simulink model "parcial2"  (R2020b)
settings: Solver=VariableStepAuto  StartTime=0.0  StopTime=30  MaxStep=1e-2  RelTol=1e-3
values from neighbouring files (symbols this model uses):
  B = 4500    [parcial.m]
  Da = 1    [parcial.m]
  fv = 1    [parcial.m]
  J = 1    [parcial.m]
  J1 = 0.5    [parcial.m]
  Ja = 1    [parcial.m]
  K = a2*(5+4*M)    (= 0.316831683168)    [parcial.m]
  K1 = 1000    [parcial.m]
  K2 = 5000    [parcial.m]
  K3 = 1200    [parcial.m]
  Kb = 1    [parcial.m]
  M = (12/a1-5)/4    (= -0.136138613861)    [parcial.m]
  M1 = 2    [parcial.m]
  M2 = 3    [parcial.m]
  N1 = 10    [parcial.m]
  N2 = 20    [parcial.m]
  R = 2    [parcial.m]
  R1 = 0.3    [parcial.m]
  R2 = 0.025    [parcial.m]
  Ra = 1    [parcial.m]
undefined symbols (not defined in the file or in its folder): Ki
settings Model: Creator=Acer  LastModifiedBy=Acer

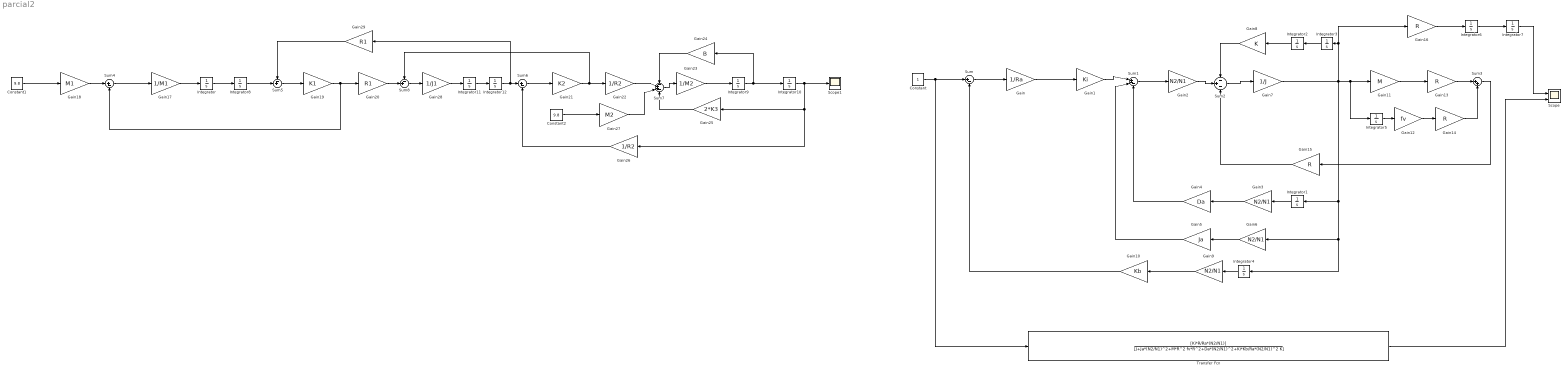
== system parcial2 ==
  Constant : Constant
  Constant1 : Constant  Value=9.8
  Constant2 : Constant  Value=9.8
  Gain : Gain  Gain=1/Ra
  Gain1 : Gain  Gain=Ki
  Gain10 : Gain  Gain=Kb
  Gain11 : Gain  Gain=M
  Gain12 : Gain  Gain=fv
  Gain{13..16} (4 alike) : Gain  Gain=R
  Gain17 : Gain  Gain=1/M1
  Gain18 : Gain  Gain=M1
  Gain19 : Gain  Gain=K1
  Gain{2..3,6,9} (4 alike) : Gain  Gain=N2/N1
  Gain20 : Gain  Gain=R1
  Gain21 : Gain  Gain=K2
  Gain22 : Gain  Gain=1/R2
  Gain23 : Gain  Gain=1/M2
  Gain24 : Gain  Gain=B
  Gain25 : Gain  Gain=2*K3
  Gain26 : Gain  Gain=1/R2
  Gain27 : Gain  Gain=M2
  Gain28 : Gain  Gain=1/J1
  Gain29 : Gain  Gain=R1
  Gain4 : Gain  Gain=Da
  Gain5 : Gain  Gain=Ja
  Gain7 : Gain  Gain=1/J
  Gain8 : Gain  Gain=K
  Integrator{,1..12} (13 alike) : Integrator
  Scope : Scope  NumInputPorts=2
  Scope1 : Scope
  Sum : Sum  Inputs=|+-
  Sum1 : Sum  Inputs=|+--
  Sum2 : Sum  Inputs=-+-
  Sum3 : Sum  Inputs=|++
  Sum4 : Sum  Inputs=|+-
  Sum5 : Sum  Inputs=-+|
  Sum6 : Sum  Inputs=|+-
  Sum7 : Sum  Inputs=-++-
  Sum8 : Sum  Inputs=-+|
  Transfer Fcn : TransferFcn  Numerator=[Ki*R/Ra*(N2/N1)]  Denominator=[J+Ja*(N2/N1)^2+M*R^2 fv*R^2+Da*(N2/N1)^2+Ki*Kb/Ra*(N2/N1)^2 K]
  wires:
  Sum/1 -> Gain/1
  Gain/1 -> Gain1/1
  Gain1/1 -> Sum1/1
  Sum1/1 -> Gain2/1
  Gain2/1 -> Sum2/2
  Integrator1/1 -> Gain3/1
  Gain3/1 -> Gain4/1
  Gain4/1 -> Sum1/3
  Gain6/1 -> Gain5/1
  Gain5/1 -> Sum1/2
  Sum2/1 -> Gain7/1
  Gain8/1 -> Sum2/1
  Integrator2/1 -> Gain8/1
  Integrator3/1 -> Integrator2/1
  Gain7/1 -> Gain16/1, Integrator3/1, Integrator5/1, Gain11/1, Integrator4/1, Gain6/1, Integrator1/1
  Integrator4/1 -> Gain9/1
  Gain9/1 -> Gain10/1
  Gain10/1 -> Sum/2
  Integrator5/1 -> Gain12/1
  Gain11/1 -> Gain13/1
  Gain12/1 -> Gain14/1
  Gain13/1 -> Sum3/1
  Gain14/1 -> Sum3/2
  Sum3/1 -> Gain15/1
  Gain15/1 -> Sum2/3
  Constant/1 -> Transfer Fcn/1, Sum/1
  Transfer Fcn/1 -> Scope/2
  Gain16/1 -> Integrator6/1
  Integrator6/1 -> Integrator7/1
  Integrator7/1 -> Scope/1
  Sum4/1 -> Gain17/1
  Gain18/1 -> Sum4/1
  Constant1/1 -> Gain18/1
  Gain17/1 -> Integrator/1
  Integrator/1 -> Integrator8/1
  Integrator8/1 -> Sum5/2
  Sum5/1 -> Gain19/1
  Gain19/1 -> Gain20/1, Sum4/2
  Sum6/1 -> Gain21/1
  Gain21/1 -> Gain22/1, Sum8/1
  Gain22/1 -> Sum7/2
  Sum7/1 -> Gain23/1
  Gain23/1 -> Integrator9/1
  Gain24/1 -> Sum7/1
  Integrator9/1 -> Integrator10/1, Gain24/1
  Integrator10/1 -> Scope1/1, Gain26/1, Gain25/1
  Gain26/1 -> Sum6/2
  Gain25/1 -> Sum7/4
  Constant2/1 -> Gain27/1
  Gain27/1 -> Sum7/3
  Gain20/1 -> Sum8/2
  Sum8/1 -> Gain28/1
  Gain28/1 -> Integrator11/1
  Integrator11/1 -> Integrator12/1
  Integrator12/1 -> Gain29/1, Sum6/1
  Gain29/1 -> Sum5/1
